simulink model "Simulink_PID"  (R2016a)
settings: Solver=FixedStepAuto  StartTime=0  StopTime=30.0  FixedStep=0.001  RelTol=1e-3
values from neighbouring files (symbols this model uses):
  k1 = 1 - a0    [Controllable.m]    (also in ControllableV1.m = 1 + a0; ControllableV2.m = Ccoef_poly(1) + a0)
  k2 = -4 - a1    [Controllable.m]    (also in ControllableV1.m = 4 + a1; ControllableV2.m = Ccoef_poly(2) + a1)
undefined symbols (not defined in the file or in its folder): c2, Ds, J2, khw
libraries: simulink x6
settings Model: Creator=om_kha  LastModifiedBy=om_kha

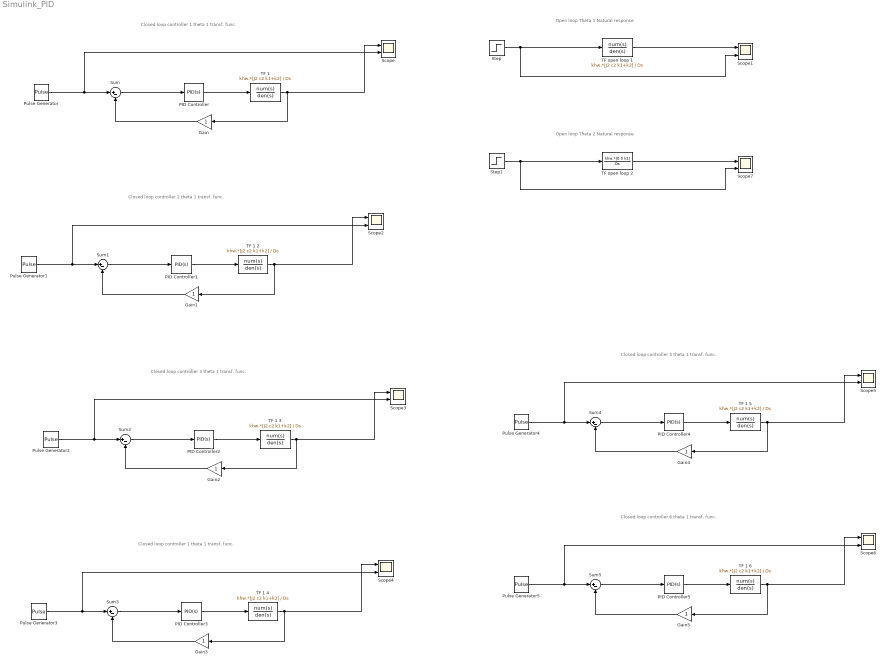
== system Simulink_PID ==
  note: Closed loop controller 1 theta 1 transf. func.
  note: Open loop Theta 1 Natural response
  note: Closed loop controller 2 theta 1 transf. func.
  note: Closed loop controller 3 theta 1 transf. func.
  note: Closed loop controller 1 theta 1 transf. func.
  note: Closed loop controller 5 theta 1 transf. func.
  note: Closed loop controller 6 theta 1 transf. func.
  note: Open loop Theta 2 Natural response
  Gain{,1..5} (6 alike) : Gain
  PID Controller{,1..5} (6 alike) : simulink/Continuous/PID Controller  Controller=PID  TimeDomain=Continuous-time  SampleTime=-1  IntegratorMethod=Forward Euler  FilterMethod=Forward Euler  Form=Parallel  UseFilter=on  ControllerParametersSource=internal  P=0.0246  I=0.74452  D=2.1517e-04  N=100  InitialConditionSource=internal  InitialConditionForIntegrator=0  InitialConditionForFilter=0  ExternalReset=none  LimitOutput=off  UpperSaturationLimit=inf  LowerSaturationLimit=-inf  LinearizeAsGain=on  AntiWindupMode=none  Kb=1  TrackingMode=off  Kt=1  PParamMin=[]  PParamMax=[]  IParamMin=[]  IParamMax=[]  DParamMin=[]  DParamMax=[]  NParamMin=[]  NParamMax=[]  KbParamMin=[]  KbParamMax=[]  KtParamMin=[]  KtParamMax=[]  POutMin=[]  POutMax=[]  IOutMin=[]  IOutMax=[]  DOutMin=[]  DOutMax=[]  NOutMin=[]  NOutMax=[]  KbOutMin=[]  KbOutMax=[]  KtOutMin=[]  KtOutMax=[]  IntegratorOutMin=[]  IntegratorOutMax=[]  FilterOutMin=[]  FilterOutMax=[]  SumOutMin=[]  SumOutMax=[]  SumI1OutMin=[]  SumI1OutMax=[]  SumI2OutMin=[]  SumI2OutMax=[]  SumI3OutMin=[]  SumI3OutMax=[]  SumDOutMin=[]  SumDOutMax=[]  SaturationOutMin=[]  SaturationOutMax=[]  IntegratorContinuousStateAttributes=''  IntegratorStateMustResolveToSignalObject=off  IntegratorRTWStateStorageClass=Auto  FilterContinuousStateAttributes=''  FilterStateMustResolveToSignalObject=off  FilterRTWStateStorageClass=Auto  DifferentiatorICPrevScaledInput=0  DifferentiatorOutMin=[]  DifferentiatorOutMax=[]
  Pulse Generator{,1..5} (6 alike) : DiscretePulseGenerator  PulseType=Time based  Period=10  PulseWidth=50
  Scope{,1..7} (8 alike) : Scope  NumInputPorts=2
  Step : Step  Time=5  Before=50  After=0  SampleTime=0
  Step1 : Step  Time=5  Before=50  After=0  SampleTime=0
  Sum{,1..5} (6 alike) : Sum  Inputs=|+-
  TF 1 {,2..6} (6 alike) : TransferFcn  Numerator=khw.*[J2 c2 k1+k2]  Denominator=Ds  ContinuousStateAttributes='tf1_plant'
  TF open loop 1 : TransferFcn  Numerator=khw.*[J2 c2 k1+k2]  Denominator=Ds  ContinuousStateAttributes='tf1_plant'
  TF open loop 2 : TransferFcn  Numerator=khw.*[0 0 k1]  Denominator=Ds  ContinuousStateAttributes='tf2_plant'
  wires:
  PID Controller/1 -> "TF 1 "/1
  "TF 1 "/1 -> Scope/1, Gain/1
  Pulse Generator/1 -> Scope/2, Sum/1
  Sum/1 -> PID Controller/1
  Gain/1 -> Sum/2
  TF open loop 1/1 -> Scope1/1
  Step/1 -> Scope1/2, TF open loop 1/1
  PID Controller1/1 -> TF 1 2/1
  TF 1 2/1 -> Scope2/1, Gain1/1
  Pulse Generator1/1 -> Scope2/2, Sum1/1
  Sum1/1 -> PID Controller1/1
  Gain1/1 -> Sum1/2
  PID Controller2/1 -> TF 1 3/1
  TF 1 3/1 -> Scope3/1, Gain2/1
  Pulse Generator2/1 -> Scope3/2, Sum2/1
  Sum2/1 -> PID Controller2/1
  Gain2/1 -> Sum2/2
  PID Controller3/1 -> TF 1 4/1
  TF 1 4/1 -> Scope4/1, Gain3/1
  Pulse Generator3/1 -> Scope4/2, Sum3/1
  Sum3/1 -> PID Controller3/1
  Gain3/1 -> Sum3/2
  PID Controller4/1 -> TF 1 5/1
  TF 1 5/1 -> Scope5/1, Gain4/1
  Pulse Generator4/1 -> Scope5/2, Sum4/1
  Sum4/1 -> PID Controller4/1
  Gain4/1 -> Sum4/2
  PID Controller5/1 -> TF 1 6/1
  TF 1 6/1 -> Scope6/1, Gain5/1
  Pulse Generator5/1 -> Scope6/2, Sum5/1
  Sum5/1 -> PID Controller5/1
  Gain5/1 -> Sum5/2
  TF open loop 2/1 -> Scope7/1
  Step1/1 -> Scope7/2, TF open loop 2/1
